simulink model "QuadLinearization"  (R2024a)
settings: Solver=VariableStepAuto  StartTime=0.0  StopTime=10.0  RelTol=1e-3
values from neighbouring files (symbols this model uses):
  allocation_matrix = [0   0.5    0.25 0.25 ... (first row only)    [quad_data.m]
  b = data(6)    [quad_data.m]
  d = data(7)    [quad_data.m]
  g = data(5)    [quad_data.m]
  L = data(8)    [quad_data.m]
  m = data(1)    [quad_data.m]
  motors_no = 4    [quad_data.m]
  omega_max = sqrt(2)*omega_nom    [quad_data.m]
  omega_nom = sqrt((m*g)/(motors_no*b))    [quad_data.m]
undefined symbols (not defined in the file or in its folder): sigbuilder_block
libraries: shared6dof x1
settings Model: Creator=Mustafa Taha  LastModifiedBy=Mustafa Taha

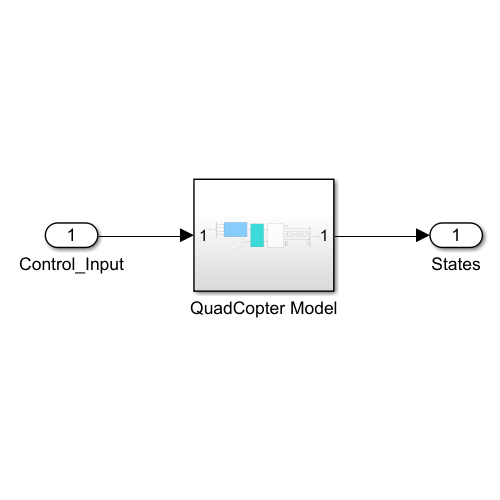
[thumbnail: Simulink's stored preview of the top-level diagram]
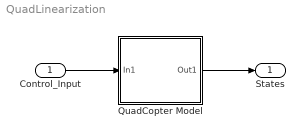
== system QuadLinearization ==
  Control_Input : Inport
  QuadCopter Model : Subsystem
  States : Outport
  wires:
  Control_Input/1 -> QuadCopter Model/1(In1)
  QuadCopter Model/1(Out1) -> States/1

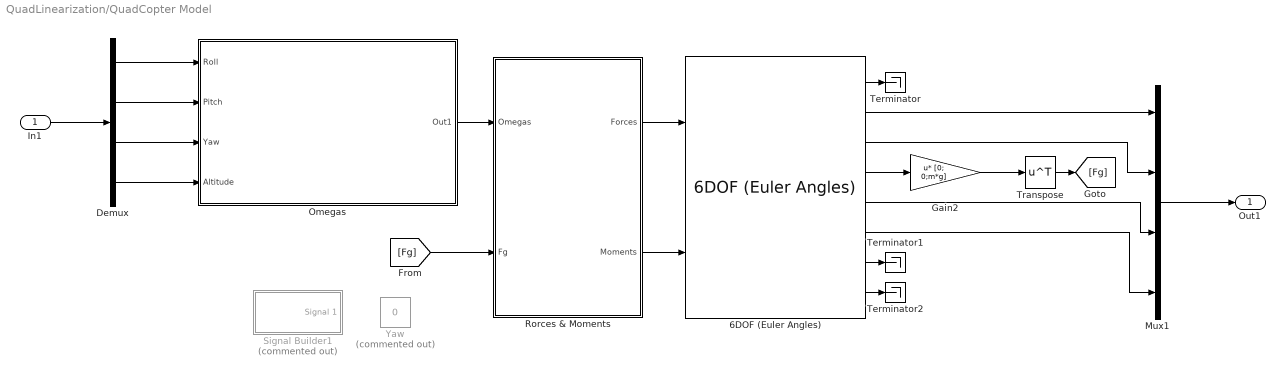
== system QuadLinearization/QuadCopter Model ==
  In1 : Inport
  6DOF (Euler Angles) : shared6dof/6DOF (Euler Angles)  units=Metric (MKS)  mtype=Fixed  rep=Euler Angles  xme_0=[0 0 -1]  Vm_0=[0 0 0]  eul_0=[0 0 0]  pm_0=[0 0 0]  mass_0=m  mass_e=0.5  mass_f=2.0  inertia=I  inertia_e=eye(3)  inertia_f=2*eye(3)  k_quat=1.0  vre_flag=on  abi_flag=off  aMode=0  xme_statename=''  Vm_statename=''  eul_statename=''  quat_statename=''  pm_statename=''  mass_statename=''
  Demux : Demux
  Gain2 : Gain  Gain=[0; 0;m*g]  Multiplication=Matrix(u*K)
  Mux1 : Mux
  Omegas : Subsystem
  Rorces & Moments : Subsystem
  Signal Builder1 : Subsystem  Tag=STV Subsys  Commented=on  LoadFcn=sigbuilder_block('load');  StartFcn=sigbuilder_block('start');  StopFcn=sigbuilder_block('stop');  ClipboardFcn=sigbuilder_block('clipboard');  mask(Sigbuilder block){tuvar=[0:10]}
      mask help: Simulink:masks:SigbuilderBlock_MD
      mask init:
      | if ~strcmp(get_param(bdroot(gcbh),'SimulationStatus'),'stopped') tuvar = sigbuilder_block('maskInit'); end
      settings: CopyFcn=sigbuilder_block('copy');  DeleteFcn=sigbuilder_block('delete');  ModelCloseFcn=sigbuilder_block('modelClose');  PreSaveFcn=sigbuilder_block('preSave');  PauseFcn=sigbuilder_block('pause');  ContinueFcn=sigbuilder_block('continue');  NameChangeFcn=sigbuilder_block('namechange');  OpenFcn=sigbuilder_block('open',[394.2 60 550.8 400.2 ]);  CloseFcn=sigbuilder_block('close');
      mask Display: plot(0, 0, 100, 100,[2, 2, 32, 32, 2], [68, 8, 8, 68, 68],[32, 2], [38, 38], [32, 19, 2],[53, 60, 44], [32, 17, 17, 2],[16, 16, 31, 31]);txt = getActiveGroup(gcbh);text(2, 100, txt,'verticalAlignment', 'top');
  Terminator : Terminator
  Terminator1 : Terminator
  Terminator2 : Terminator
  Transpose : Math  Operator=transpose
  Yaw : Constant  Commented=on  Value=0
  Out1 : Outport
  wires:
  6DOF (Euler Angles)/6 -> Mux1/4
  6DOF (Euler Angles)/2 -> Mux1/1
  Transpose/1 -> [Fg]
  6DOF (Euler Angles)/3 -> Mux1/2
  Omegas/1(Out1) -> Rorces & Moments/1(Omegas)
  Demux/2 -> Omegas/2("Pitch ")
  6DOF (Euler Angles)/1 -> Terminator/1
  Mux1/1 -> Out1/1
  6DOF (Euler Angles)/7 -> Terminator1/1
  6DOF (Euler Angles)/4 -> Gain2/1
  6DOF (Euler Angles)/8 -> Terminator2/1
  Demux/3 -> Omegas/3("Yaw ")
  In1/1 -> Demux/1
  [Fg] -> Rorces & Moments/2(Fg)
  Demux/1 -> Omegas/1("Roll ")
  Rorces & Moments/1(Forces) -> 6DOF (Euler Angles)/1
  6DOF (Euler Angles)/5 -> Mux1/3
  Gain2/1 -> Transpose/1
  Rorces & Moments/2(Moments) -> 6DOF (Euler Angles)/2
  Demux/4 -> Omegas/4("Altitude ")

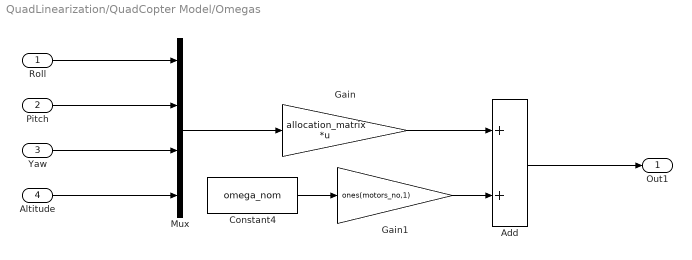
== system QuadLinearization/QuadCopter Model/Omegas ==
  "Roll " : Inport
  "Pitch " : Inport  Port=2
  "Yaw " : Inport  Port=3
  "Altitude " : Inport  Port=4
  Add : Sum
  Constant4 : Constant  Value=omega_nom
  Gain : Gain  Gain=allocation_matrix  Multiplication=Matrix(K*u)
  Gain1 : Gain  Gain=ones(motors_no,1)
  Mux : Mux
  Out1 : Outport
  wires:
  Mux/1 -> Gain/1
  "Yaw "/1 -> Mux/3
  Constant4/1 -> Gain1/1
  "Roll "/1 -> Mux/1
  "Pitch "/1 -> Mux/2
  Gain/1 -> Add/1
  "Altitude "/1 -> Mux/4
  Gain1/1 -> Add/2
  Add/1 -> Out1/1

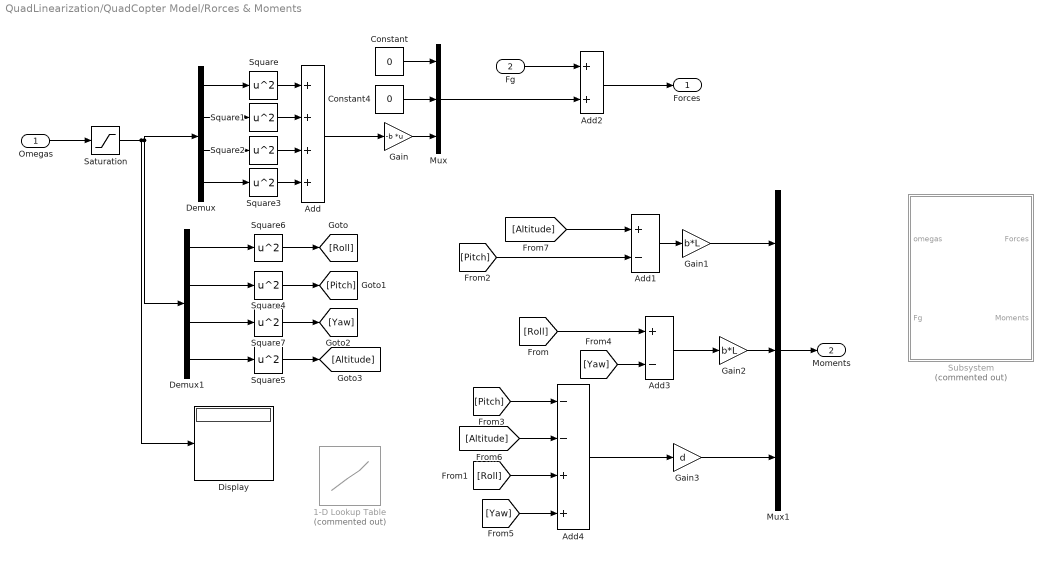
== system QuadLinearization/QuadCopter Model/Rorces & Moments ==
  Omegas : Inport
  Fg : Inport  Port=2
  1-D Lookup Table : Lookup_n-D  Commented=on  NumberOfTableDimensions=1  BreakpointsForDimension1=[0 omega_nom sqrt(2)*omega_nom]  Table=[-1 0 1]  InternalRulePriority=Speed  RndMeth=Simplest
  Add : Sum  Inputs=++++
  Add1 : Sum  Inputs=+-
  Add2 : Sum
  Add3 : Sum  Inputs=+-
  Add4 : Sum  Inputs=--++
  Constant : Constant  Value=0
  Constant4 : Constant  Value=0
  Demux : Demux
  Demux1 : Demux
  Display : Display
  Gain : Gain  Gain=-b  Multiplication=Matrix(K*u)
  Gain1 : Gain  Gain=b*L
  Gain2 : Gain  Gain=b*L
  Gain3 : Gain  Gain=d
  Mux : Mux  Inputs=3
  Mux1 : Mux  Inputs=3
  Saturation : Saturate  UpperLimit=omega_max
  Square{,1..7} (8 alike) : Math  Operator=square
  Subsystem : Subsystem  Commented=on
  Forces : Outport
  Moments : Outport  Port=2
  wires:
  Add/1 -> Gain/1
  Square2/1 -> Add/3
  Square3/1 -> Add/4
  Square/1 -> Add/1
  Demux/3 -> Square2/1
  Square1/1 -> Add/2
  Demux/2 -> Square1/1
  Fg/1 -> Add2/1
  Mux/1 -> Add2/2
  Demux/4 -> Square3/1
  Gain/1 -> Mux/3
  Add2/1 -> Forces/1
  Demux/1 -> Square/1
  Constant/1 -> Mux/1
  Constant4/1 -> Mux/2
  Demux1/2 -> Square4/1
  Demux1/4 -> Square5/1
  Demux1/1 -> Square6/1
  Demux1/3 -> Square7/1
  Add1/1 -> Gain1/1
  Add3/1 -> Gain2/1
  Add4/1 -> Gain3/1
  Gain2/1 -> Mux1/2
  Gain1/1 -> Mux1/1
  Gain3/1 -> Mux1/3
  Mux1/1 -> Moments/1
  Square6/1 -> [Roll]
  [Roll] -> Add3/1
  [Roll] -> Add4/3
  Square4/1 -> [Pitch]
  [Pitch] -> Add1/2
  [Pitch] -> Add4/1
  [Yaw] -> Add4/4
  [Yaw] -> Add3/2
  Square7/1 -> [Yaw]
  Square5/1 -> [Altitude]
  [Altitude] -> Add4/2
  [Altitude] -> Add1/1
  Saturation/1 -> Demux/1, Demux1/1, Display/1
  Omegas/1 -> Saturation/1

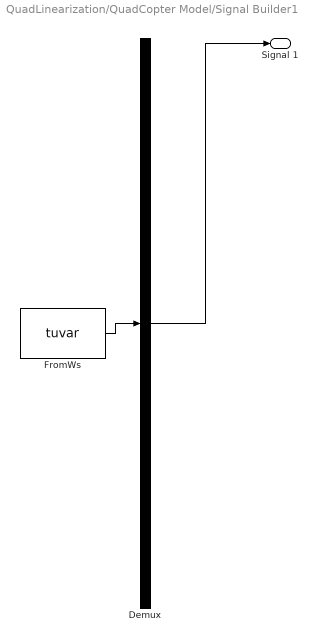
== system QuadLinearization/QuadCopter Model/Signal Builder1 ==
  Demux : Demux  Tag=STV Demux  Outputs=1
      settings: DisplayOption=none
  FromWs : FromWorkspace  Tag=STV FromWs  VariableName=tuvar
      SigBuilderData=|
      | common.afterFinalStr = 'Extrapolate'
      | common.sampleTime = 0
      | dataSet.timeRange = [0 10]
      | dataSet.name = 'Group 1'
      | sbobj.Groups.Name = 'Group 1'
      | sbobj.Groups.Signals.Name = 'Signal 1'
      | sbobj.Groups.Signals.XData = [0 4 4 6 6 10]
      | sbobj.Groups.Signals.YData = [0 0.06 5 5 0 0]
  Signal 1 : Outport  Tag=STV Outport
  wires:
  FromWs/1 -> Demux/1
  Demux/1 -> Signal 1/1

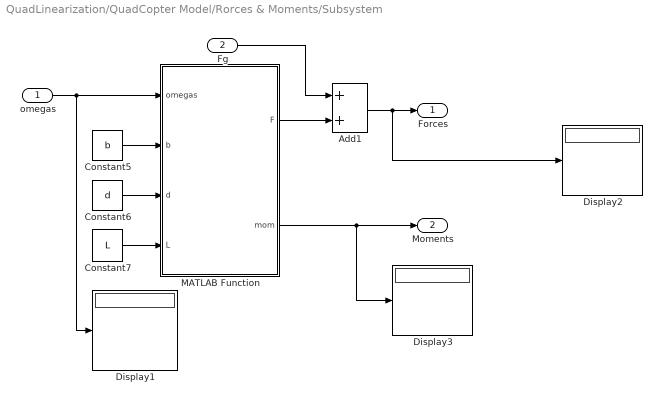
== system QuadLinearization/QuadCopter Model/Rorces & Moments/Subsystem ==
  omegas : Inport
  Fg : Inport  Port=2
  Add1 : Sum
  Constant5 : Constant  Value=b
  Constant6 : Constant  Value=d
  Constant7 : Constant  Value=L
  Display1 : Display
  Display2 : Display
  Display3 : Display
  MATLAB Function : MATLAB Function  TreatAsAtomicUnit=on
  Forces : Outport
  Moments : Outport  Port=2
  wires:
  Constant6/1 -> MATLAB Function/3(d)
  MATLAB Function/1(F) -> Add1/2
  Add1/1 -> Display2/1, Forces/1
  Fg/1 -> Add1/1
  Constant7/1 -> MATLAB Function/4(L)
  Constant5/1 -> MATLAB Function/2(b)
  MATLAB Function/2(mom) -> Display3/1, Moments/1
  omegas/1 -> MATLAB Function/1(omegas), Display1/1

== matlab function QuadLinearization/QuadCopter Model/Rorces & Moments/Subsystem/MATLAB Function ==
  data: omegas input; F output; b input; d input; L input; mom output
function [F,mom] = fcn(omegas,b,d,L)
w1= omegas(1);
w2= omegas(2);
w3= omegas(3);
w4= omegas(4);

%deltas (roll,pitch,yaw,thrust)
F = [0 0 -b*(w1^2 + w2^2 +w3^2 + w4^2)];
mom = [b*L*(w4^2-w2^2)...
    b*L*(w1^2-w3^2)...
    d*(-w2^2-w4^2+w1^2+w3^2)];
